simulink model "Loop_detailed_model_comp_cc_vccc_v12"  (R2013a)
settings: Solver=ode45  SolverMode=SingleTasking  StartTime=0.0  StopTime=8e-3  FixedStep=FS/50  MaxStep=1e-4  RelTol=1e-3
InitFcn:
  | %%%%%%  set scope time range
  | T_STOP=str2num(get_param(gcs,'StopTime'));
  | if numel(T_STOP) > 1
  |    T_STOP=T_STOP(2);
  | else
  |    T_STOP=T_STOP(1);
  | end
  | T_STOP=num2str(T_STOP);
  | 
  | %%%%%%  set scope time range in system @init_callback_fct
  | T_STOP=num2str(str2num(get_param(gcs,'StopTime')));
  | 
  | childs = allchild(0);
  | sol=strfind(upper(get(allchild(0),'Tag')),'VIEWER_PARAMETERS');
  | 
  | if iscell(sol)
  |    ind=find(~cellfun(@isempty, strfind(upper(get(allchild(0),'Tag')),'VIEWER_PARAMETERS')));
  | else
  |    ind=sol;
  | end
  | %ind=find(~cellfun(@isempty, {strfind(upper(get(allchild(0),'Tag')),'VIEWER_PARAMETERS'),[]}))
  | if ~isempty(ind)
  |    for k=1:length(childs(ind))
  |       set_param(getfield(get(childs(ind(k)),'UserData'),'block'),'TimeRange', T_STOP);
  | %      get_param(getfield(get(childs(ind(k)),'UserData'),'block'),'TimeRange');
  | %    set_param(getfield(get(childs(ind),'UserData'),'block'),'TimeRange',T_STOP);
  | %    get_param(getfield(get(childs(ind),'UserData'),'block'),'TimeRange');
  |    end
  | else
  |     warning(sprintf('VIEWER_PARAMETERS object not found\nOpen the config dialog by hand for the first sim start'))
  | end
undefined symbols (not defined in the file or in its folder): FS, Lc, Rc, Rsh, T1
libraries: simulink x1
settings Model: BufferReuse=off  Creator=mainster  LastModifiedBy=mainster
settings SolverCC: AutoInsertRateTranBlk=on
settings OptimizationCC: InlineParams=on  BufferReuse=off
settings DebuggingCC: InitInArrayFormatMsg=none
settings HardwareCC: ProdLargestAtomicInteger=Long  ProdLargestAtomicFloat=Double  ProdEndianess=LittleEndian  ProdHWDeviceType=ARM Compatible->ARM Cortex

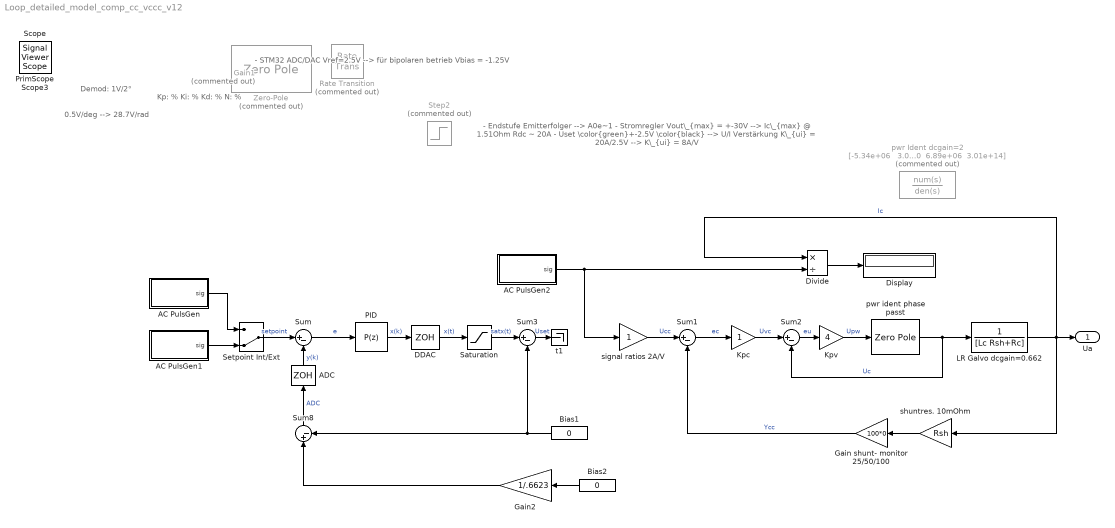
== system Loop_detailed_model_comp_cc_vccc_v12 ==
  note: - Endstufe Emitterfolger --> A0e~1
      | - Stromregler Vout\_{max} = +-30V
      |       --> Ic\_{max} @ 1.51Ohm Rdc ~ 20A
      | - Uset \color{green}+-2.5V \color{black}
      |       --> U/I Verstärkung K\_{ui} = 20A/2.5V
      |       --> K\_{ui} = 8A/V
  note: - STM32 ADC/DAC Vref=2.5V
      | --> für bipolaren betrieb Vbias = -1.25V
  note: Kp: % Ki: % Kd: % N: %
  note: 0.5V/deg --> 28.7V/rad
  note: Demod:
      | 1V/2°
  AC PulsGen : Subsystem  mask{sigp=0.3, sigpp=0, offs=0}
      mask prompts: sigp "Insert signal peak"; sigpp "or signal peak-to-peak"; offs "Insert DC offset"
      mask TypeOptions sigp: PulsGen/Amplitude
      mask Callback sigp:
      | %sigp=get_param([gcb '/PulsGen'],'Amplitude')
      | %SigVal=2*sigp
      mask TypeOptions offs: offset/Value
      mask Display:
      | %str=sprintf('%s',get(gcbh,'ModelName'));
      | port_label('output', 1, '','texmode','off')
      | %text(.05,.98,['{\fontsize{12}\it\bf' strrep(str,'_',' ') '}'],'horizontalAlignment','left','verticalAlignment','top','texmode','on')
      | %text(.5,0.95,['{\fontsize{8}A_{peak}=}'],'horizontalAlignment','center','verticalAlignment','top','texmode','on')
      | disp(sprintf('Up=%.3g\nDC=%.3g',sigp, offs))
      | %disp(['Upp=' sigpp])%, offs))
      | %sprintf('sigpp==%s',sigpp)
      | %text(.15,.05,['{\fontsize{10}\itmechanics}'],'horizontalAlignment','left','verticalAlignment','bottom','texmode','on')
  AC PulsGen1 : Subsystem  mask{sigp=1, sigpp=0, offs=0}
      mask prompts: sigp "Insert signal peak"; sigpp "or signal peak-to-peak"; offs "Insert DC offset"
      mask TypeOptions sigp: PulsGen/Amplitude
      mask Callback sigp:
      | %sigp=get_param([gcb '/PulsGen'],'Amplitude')
      | %SigVal=2*sigp
      mask TypeOptions offs: offset/Value
      mask Display:
      | %str=sprintf('%s',get(gcbh,'ModelName'));
      | port_label('output', 1, '','texmode','off')
      | %text(.05,.98,['{\fontsize{12}\it\bf' strrep(str,'_',' ') '}'],'horizontalAlignment','left','verticalAlignment','top','texmode','on')
      | %text(.5,0.95,['{\fontsize{8}A_{peak}=}'],'horizontalAlignment','center','verticalAlignment','top','texmode','on')
      | disp(sprintf('Up=%.3g\nDC=%.3g',sigp, offs))
      | %disp(['Upp=' sigpp])%, offs))
      | %sprintf('sigpp==%s',sigpp)
      | %text(.15,.05,['{\fontsize{10}\itmechanics}'],'horizontalAlignment','left','verticalAlignment','bottom','texmode','on')
  AC PulsGen2 : Subsystem  mask{sigp=1, sigpp=0, offs=0}
      mask prompts: sigp "Insert signal peak"; sigpp "or signal peak-to-peak"; offs "Insert DC offset"
      mask TypeOptions sigp: PulsGen/Amplitude
      mask Callback sigp:
      | %sigp=get_param([gcb '/PulsGen'],'Amplitude')
      | %SigVal=2*sigp
      mask TypeOptions offs: offset/Value
      mask Display:
      | %str=sprintf('%s',get(gcbh,'ModelName'));
      | port_label('output', 1, '','texmode','off')
      | %text(.05,.98,['{\fontsize{12}\it\bf' strrep(str,'_',' ') '}'],'horizontalAlignment','left','verticalAlignment','top','texmode','on')
      | %text(.5,0.95,['{\fontsize{8}A_{peak}=}'],'horizontalAlignment','center','verticalAlignment','top','texmode','on')
      | disp(sprintf('Up=%.3g\nDC=%.3g',sigp, offs))
      | %disp(['Upp=' sigpp])%, offs))
      | %sprintf('sigpp==%s',sigpp)
      | %text(.15,.05,['{\fontsize{10}\itmechanics}'],'horizontalAlignment','left','verticalAlignment','bottom','texmode','on')
  ADC : ZeroOrderHold  SampleTime=FS
  Bias1 : Constant  Value=0  OutDataTypeStr=double  SampleTime=-1
  Bias2 : Constant  Value=0  OutDataTypeStr=double  SampleTime=-1
  DDAC : ZeroOrderHold  SampleTime=FS
      settings: AttributesFormatString=%<SampleTime>
  Display : Display
  Divide : Product  Inputs=*/
  Gain shunt- monitor 25/50/100 : Gain  Gain=100*0
  Gain1 : Gain  Commented=on  Gain=2
  Gain2 : Gain  Gain=1/.6623
  Kpc : Gain
  Kpv : Gain  Gain=4
  LR Galvo dcgain=0.662 : TransferFcn  Numerator=1  Denominator=[Lc Rsh+Rc]
  "PID " : simulink/Continuous/PID Controller  Controller=P  TimeDomain=Discrete-time  SampleTime=-1  IntegratorMethod=Forward Euler  FilterMethod=Forward Euler  Form=Parallel  P=5  I=8149.05991185772  D=9.0248898483108e-05  N=10930.7783722874  InitialConditionSource=internal  InitialConditionForIntegrator=0  InitialConditionForFilter=0  ExternalReset=none  LimitOutput=off  UpperSaturationLimit=1.25  LowerSaturationLimit=-1.25  LinearizeAsGain=on  AntiWindupMode=clamping  Kb=1  TrackingMode=off  Kt=1  PParamMin=[]  PParamMax=[]  IParamMin=[]  IParamMax=[]  DParamMin=[]  DParamMax=[]  NParamMin=[]  NParamMax=[]  KbParamMin=[]  KbParamMax=[]  KtParamMin=[]  KtParamMax=[]  POutMin=[]  POutMax=[]  IOutMin=[]  IOutMax=[]  DOutMin=[]  DOutMax=[]  NOutMin=[]  NOutMax=[]  KbOutMin=[]  KbOutMax=[]  KtOutMin=[]  KtOutMax=[]  IntegratorOutMin=[]  IntegratorOutMax=[]  FilterOutMin=[]  FilterOutMax=[]  SumOutMin=[]  SumOutMax=[]  SumI1OutMin=[]  SumI1OutMax=[]  SumI2OutMin=[]  SumI2OutMax=[]  SumI3OutMin=[]  SumI3OutMax=[]  SumDOutMin=[]  SumDOutMax=[]  SaturationOutMin=[]  SaturationOutMax=[]  IntegratorContinuousStateAttributes=''  IntegratorStateMustResolveToSignalObject=off  IntegratorRTWStateStorageClass=Auto  FilterContinuousStateAttributes=''  FilterStateMustResolveToSignalObject=off  FilterRTWStateStorageClass=Auto
      settings: AttributesFormatString=UpLim=%<UpperSaturationLimit>\nLoLim=%<LowerSaturationLimit>\nKp=%<P>
  Rate Transition : RateTransition  Commented=on  OutPortSampleTime=FS
  Saturation : Saturate  UpperLimit=1.25  LowerLimit=-1.25
      settings: AttributesFormatString=Up_lim=%<UpperLimit>\nLo_lim=%<LowerLimit>
  Setpoint Int/Ext : ManualSwitch  CurrentSetting=0
  Step2 : Step  Commented=on  Time=0  After=1.25  SampleTime=0
      settings: AttributesFormatString=Time:%<Time>\nAmp:%<After>
  Sum{,1..3,8} (5 alike) : Sum  Inputs=|+-
  Zero-Pole : ZeroPole  Commented=on  Zeros=[]  Poles=[-1/T1 -1/T1]  Gain=(1/T1)^2
  pwr Ident dcgain=2 : TransferFcn  Commented=on  Numerator="[-5.34e+06   3.00e+14]"  Denominator="[1.00e+00  6.89e+06  3.01e+14]"
  pwr ident phase passt : ZeroPole  Zeros=[]  Poles=[-7.2010 -0.0385]*1e9  Gain=2.76e17
  shuntres. 10mOhm : Gain  Gain=Rsh
  signal ratios 2A/V : Gain
  t1 : Terminator
  Ua : Outport
  PrimScope : SignalViewerScope  IOType=viewer  NumInputPorts=6  RefreshTime=0.035000
      settings: ShowLegends=on  TimeRange=0.008  YMin=-1~-2~-2~-1~-1~-2  YMax=1~2~2~1~1~2
  Scope : SignalViewerScope  IOType=viewer  RefreshTime=0.035000
  Scope3 : SignalViewerScope  IOType=viewer  ZoomMode=yonly  RefreshTime=0.035000
      settings: YMin=1  YMax=3  SaveName=ScopeData3
  wires:
  Sum/1 -> "PID "/1  "e"
  LR Galvo dcgain=0.662/1 -> Divide/1, shuntres. 10mOhm/1, Ua/1  "Ic"
  "PID "/1 -> DDAC/1  "x(k)"
  ADC/1 -> Sum/2  "y(k)"
  Kpv/1 -> pwr ident phase passt/1  "Upw"
  pwr ident phase passt/1 -> Sum2/2, LR Galvo dcgain=0.662/1  "Uc"
  Saturation/1 -> Sum3/1  "satx(t)"
  DDAC/1 -> Saturation/1  "x(t)"
  Sum8/1 -> ADC/1  "ADC"
  Bias1/1 -> Sum3/2, Sum8/2
  Setpoint Int/Ext/1 -> Sum/1  "setpoint"
  AC PulsGen/1(sig) -> Setpoint Int/Ext/1
  AC PulsGen1/1(sig) -> Setpoint Int/Ext/2
  Gain2/1 -> Sum8/1
  Sum1/1 -> Kpc/1  "ec"
  Gain shunt- monitor 25/50/100/1 -> Sum1/2  "Ycc"
  shuntres. 10mOhm/1 -> Gain shunt- monitor 25/50/100/1
  Divide/1 -> Display/1
  signal ratios 2A/V/1 -> Sum1/1  "Ucc"
  Sum2/1 -> Kpv/1  "eu"
  Kpc/1 -> Sum2/1  "Uvc"
  AC PulsGen2/1(sig) -> Divide/2, signal ratios 2A/V/1
  Bias2/1 -> Gain2/1
  Sum3/1 -> t1/1  "Uset"

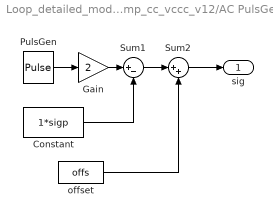
== system Loop_detailed_model_comp_cc_vccc_v12/AC PulsGen ==
  Constant : Constant  Value=1*sigp
  Gain : Gain  Gain=2  SampleTime=FS
  PulsGen : DiscretePulseGenerator  PulseType=Time based  Amplitude=sigp  Period=4e-3  PulseWidth=50  PhaseDelay=0.5e-3  SampleTime=FS
      settings: AttributesFormatString=A=%<Amplitude>\nPeri=%<Period>
  Sum1 : Sum  Inputs=|+-  SampleTime=FS
  Sum2 : Sum  Inputs=|++  SampleTime=FS
  offset : Constant  Value=offs  SampleTime=FS
  sig : Outport
  wires:
  Sum2/1 -> sig/1
  PulsGen/1 -> Gain/1
  offset/1 -> Sum2/2
  Gain/1 -> Sum1/1
  Sum1/1 -> Sum2/1
  Constant/1 -> Sum1/2

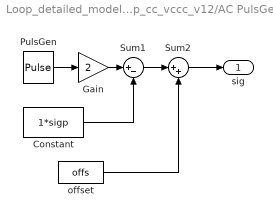
== system Loop_detailed_model_comp_cc_vccc_v12/AC PulsGen1 ==
  Constant : Constant  Value=1*sigp
  Gain : Gain  Gain=2
  PulsGen : DiscretePulseGenerator  PulseType=Time based  Amplitude=sigp  Period=4e-3  PulseWidth=50  PhaseDelay=0.5e-3  SampleTime=FS
      settings: AttributesFormatString=A=%<Amplitude>\nPeri=%<Period>
  Sum1 : Sum  Inputs=|+-
  Sum2 : Sum  Inputs=|++
  offset : Constant  Value=offs
  sig : Outport
  wires:
  Sum2/1 -> sig/1
  PulsGen/1 -> Gain/1
  offset/1 -> Sum2/2
  Gain/1 -> Sum1/1
  Sum1/1 -> Sum2/1
  Constant/1 -> Sum1/2

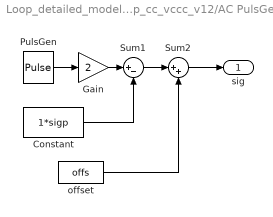
== system Loop_detailed_model_comp_cc_vccc_v12/AC PulsGen2 ==
  Constant : Constant  Value=1*sigp
  Gain : Gain  Gain=2
  PulsGen : DiscretePulseGenerator  PulseType=Time based  Amplitude=sigp  Period=4e-3  PulseWidth=50  PhaseDelay=0.5e-3  SampleTime=FS
      settings: AttributesFormatString=A=%<Amplitude>\nPeri=%<Period>
  Sum1 : Sum  Inputs=|+-
  Sum2 : Sum  Inputs=|++
  offset : Constant  Value=offs
  sig : Outport
  wires:
  Sum2/1 -> sig/1
  PulsGen/1 -> Gain/1
  offset/1 -> Sum2/2
  Gain/1 -> Sum1/1
  Sum1/1 -> Sum2/1
  Constant/1 -> Sum1/2
